simulink model "hihi_RL_prsweep"  (Simulink 8.7)
settings: Solver=VariableStepAuto  StartTime=0.0  StopTime=inf  RelTol=1e-3
settings Model: Creator=user  LastModifiedBy=Dwait
settings DataIOCC: SaveFormat=Dataset
settings DebuggingCC: UnderspecifiedInitializationDetection=Simplified  MergeDetectMultiDrivingBlocksExec=error  AllowSymbolicDim=off
settings HardwareCC: ProdBitPerPointer=64  ProdLargestAtomicFloat=Float  ProdIntDivRoundTo=Zero  ProdEndianess=LittleEndian  ProdWordSize=64  ProdHWDeviceType=Intel->x86-64 (Windows64)
settings GRTTargetCC: GeneratePreprocessorConditionals=Use local settings
settings ConfigComp: CovModelRefEnable=off
settings ConfigurationSet: Description=SimMechanics 2G

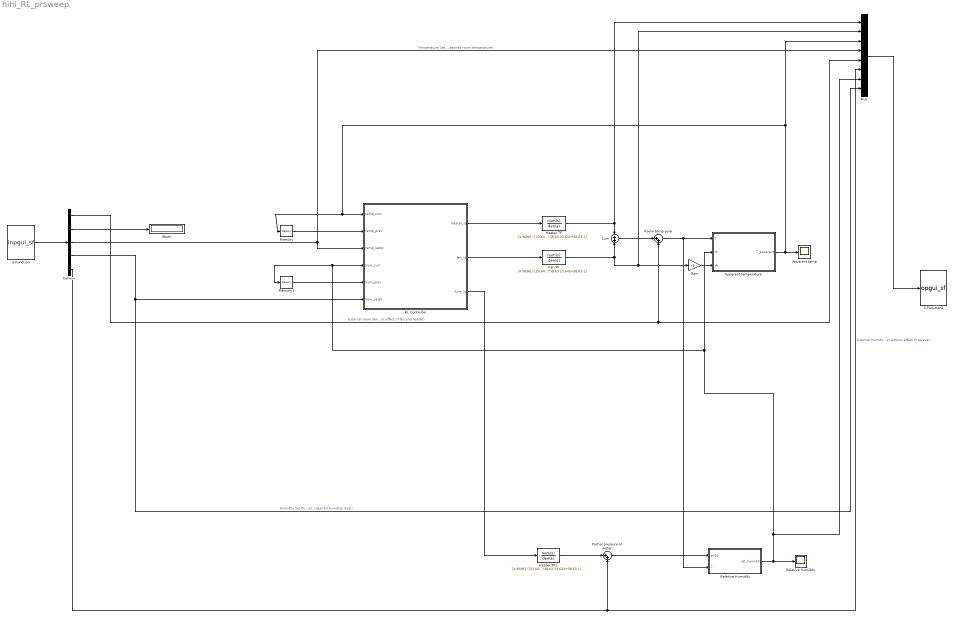
== system hihi_RL_prsweep ==
  Apparent temp : Scope
  Apparent temperature : MATLAB Function  TreatAsAtomicUnit=on
  Demux : Demux  Outputs=5
  Fan TF : TransferFcn  Numerator=[4.9696]  Denominator=[23.643*38.63 23.643+38.63 1]
  Gain : Gain  Gain=-1
  Heater TF : TransferFcn  Numerator=[4.9696]  Denominator=[23.643*38.63 23.643+38.63 1]
  Heater TF1 : TransferFcn  Numerator=[4.9696]  Denominator=[23.643*38.63 23.643+38.63 1]
  Memory : Memory
  Memory1 : Memory
  Mux : Mux  Inputs=8
  Partial pressure of water : Sum  Inputs=|++
  RL Controller : MATLAB Function  TreatAsAtomicUnit=on
  Relative Humidity : MATLAB Function  TreatAsAtomicUnit=on
  Relative humidity : Scope
  Room temp pure : Sum  Inputs=|++
  S-Function : S-Function  FunctionName=inpgui_sf  Parameters=0  SFunctionDeploymentMode=off  EnableBusSupport=off
  S-Function1 : S-Function  FunctionName=opgui_sf  Parameters=0.005  SFunctionDeploymentMode=off  EnableBusSupport=off
  Sum : Sum  Inputs=+|+
  dbutn : Display
  wires:
  S-Function/1 -> Demux/1
  Demux/2 -> dbutn/1
  Mux/1 -> S-Function1/1
  Sum/1 -> Room temp pure/1
  Demux/3 -> Mux/4, RL Controller/3(temp_setpt)  "Temperature Set Point (desired room temperature)"
  Heater TF/1 -> Mux/1, Sum/1
  RL Controller/1(heater_ip) -> Heater TF/1
  Demux/1 -> Room temp pure/2, Mux/5  "External room temperature (without effect of fan and heater)"
  RL Controller/2(fan_ip) -> Fan TF/1
  Heater TF1/1 -> Partial pressure of water/1
  Partial pressure of water/1 -> Relative Humidity/1(ph2o)
  Demux/4 -> Mux/8, RL Controller/6(hum_setpt)  "Humidity Set Point  (desired humidity level)"
  Demux/5 -> Mux/6, Partial pressure of water/2  "External humidity (without effect of sprayer)"
  Room temp pure/1 -> Relative Humidity/2(T), Apparent temperature/1(T)
  Apparent temperature/1(T_apparent) -> Mux/3, RL Controller/1(temp_curr), Memory/1, Apparent temp/1
  Fan TF/1 -> Sum/2, Gain/1, Mux/2
  Gain/1 -> Apparent temperature/3(ws)
  RL Controller/3(hum_ip) -> Heater TF1/1
  Relative Humidity/1(rel_humidity) -> Apparent temperature/2(rh), RL Controller/4(hum_curr), Memory1/1, Mux/7, Relative humidity/1
  Memory/1 -> RL Controller/2(temp_prev)
  Memory1/1 -> RL Controller/5(hum_prev)

== matlab function Relative Humidity ==
  data: ph2o input double; rel_humidity output double; T input double
function rel_humidity = relativeHumidity(ph2o,T)
P = 1013.25;        % Absolute pressure taken to be 1 atm = 1013.25 millibars

% Arden Buck equation for equilibrium vapor pressure in millibars
ph2oeq = (1.0007 + 3.46 * 10^-6 * P)*6.1121*exp(17.502*T/(240.97+T));

if (ph2o>=ph2oeq)
   rel_humidity = 100;
else
   rel_humidity = (ph2o/ph2oeq)*100;
end

== matlab function Apparent temperature ==
  data: T input double; T_apparent output double; rh input double; ws input double
%% NOTE:
%  The function works only for scalar values of T, rh and ws

function T_apparent = apparentTemp(T,rh,ws)
if(T>26.7)
    %% Heat Index calculation
    % Conversion to Fahrenheit
    T1 = 1.8*T+32;
    
    % Formula for heat index
    hIndex = - 42.379 + (2.04901523 * T1) + (10.14333127 * rh) - (0.22475541 * T1 * rh) - (6.83783 * 10^-3 * T1^2) - (5.481717 * 10^-2 * rh^2)  + (1.22874 * 10^-3 * T1^2 * rh) + (8.5282 * 10^-4 * T1 * rh^2) - (1.99 * 10^-6 * T1^2 * rh^2);
    
    % Converting result back to Celsius
    T_apparent = (hIndex-32)*5/9;
    
elseif(T<=10)
    %% Wind Chill calculation
    % Conversion to Fahrenheit, and miles per hour respectively
    T2 = 1.8*T+32;
    ws1 = 2.23694*ws;
    
    % For wind speed < 3 miles per hour (1.3 meters per sec), no wind chill effect
    if(ws1<3)
        wChill = T2;
    else
    % Formula for wind chill
    wChill = 35.74 + (0.6215 * T2) - (35.75 * ws1^0.16) + (0.4275 * T2 * ws1^0.16);
    end
     
    % Converting result back to Celsius
    T_apparent = (wChill-32)*5/9;

else
    T_apparent = T;
end

== matlab function RL Controller ==
  data: temp_curr input double; temp_prev input double; heater_ip output double; temp_setpt input double; fan_ip output double; hum_ip output double; hum_curr input double; hum_prev input double; hum_setpt input double
function [heater_ip, fan_ip, hum_ip] = fcn(temp_curr,temp_prev,temp_setpt,hum_curr,hum_prev,hum_setpt)
% The main function of the training

% Extrinsic calls to these functions which wouldn't otherwise work in
% a MATLAB function block
coder.extrinsic('BuildStateList');
coder.extrinsic('Episode_queue');
coder.extrinsic('int2str');
coder.extrinsic('num2str');
coder.extrinsic('bdroot');
coder.extrinsic('set_param');

maxepisodes = 1;

heater_ip = 0;
fan_ip = 0;
hum_ip = 0;

N = 30;     % range for temp_err
M = 30;     % range for hum_err

persistent start;
goal        = [0 0 GetTempRange(temp_setpt)];
maze        = CreateMaze(N, M);

statelist   = BuildStateList(N,M,3);  % the list of states
% [X,Y,Z] = meshgrid(0:N-1,0:M-1,0:2);
% statelist   = BuildStateList();
actionlist  = BuildActionList(); % the list of actions

nstates     = size(statelist,1);
nactions    = size(actionlist,1);

%Generate initial Population
Q           = BuildQTable(nstates,nactions); % the Qtable
Model       = BuildModel(nstates,nactions); % the Qtable

% planning steps
%p_steps     = 100;

maxsteps    = 3000;  % maximum number of steps per episode
alpha_init  = 0.8;   % initial learning rate for all (s,a) pairs
gamma       = 0.95;  % discount factor
epsilon     = 0.3;   % probability of a random act8ion selection
theta       = 0.1;   % error threshold


grafic     = true; % indicates if display the graphical interface
xpoints=zeros(1,maxepisodes);
ypoints=zeros(1,maxepisodes);

%Number of times a state has been visited (for changing alpha)
Ns = zeros(nstates,nactions);
%alpha = alpha_init.*ones(nstates,nactions);

count = 0;

% Initializing a few variables for MATLAB Coder
total_reward = 0;

for i=1:maxepisodes
    % Reducing alpha with every episode
    count = count+1;
    alpha = alpha_init / count;
    start = GetState(temp_prev,temp_setpt,hum_prev,hum_setpt);
    
    [ total_reward,steps,Q,Model,Ns,heater_ip, fan_ip, hum_ip ] = Episode_queue( maxsteps, Q,Model , alpha, Ns, gamma,epsilon,theta,statelist,actionlist,grafic,maze,start,goal,heater_ip, fan_ip, hum_ip, temp_curr, hum_curr );

    disp(['Espisode: ',int2str(i),'  Steps:',int2str(steps),'  Reward:',num2str(total_reward),' epsilon: ',num2str(epsilon)])
    
    epsilon = epsilon*0.9;
    
    % Reducing alpha for visited states
    % alpha(Ns>1) = alpha(Ns>1) ./ Ns(Ns>1);
    
    
    xpoints(i)=i-1;
    ypoints(i)=steps;
    subplot(2,1,2);
    plot(xpoints(1:i),ypoints(1:i))
    title(['Episode: ',int2str(i),' epsilon: ',num2str(epsilon)])
    
    drawnow
    
    if (i>2000000)
        grafic=true;
    end
    
    set_param(bdroot,'SimulationCommand','pause');
    set_param
    set_param(bdroot,'SimulationCommand','start');

end
